simulink model "SpringMass_Model_SDomain"  (R2020a)
settings: Solver=VariableStepAuto  StartTime=0.0  StopTime=10  MaxStep=0.05  RelTol=1e-3
values from neighbouring files (symbols this model uses):
  b = 1.8    [SpringMass_mScript_SDomain.m]    (also in SpringMass_mScript_TDomain.m = 2)
  F = 10    [SpringMass_mScript_SDomain.m]    (also in SpringMass_mScript_TDomain.m)
  k = 10    [SpringMass_mScript_SDomain.m]    (also in SpringMass_mScript_TDomain.m = 20)
  M = 1    [SpringMass_mScript_SDomain.m]    (also in SpringMass_mScript_TDomain.m)
settings Model: Creator=alexd  LastModifiedBy=alexd

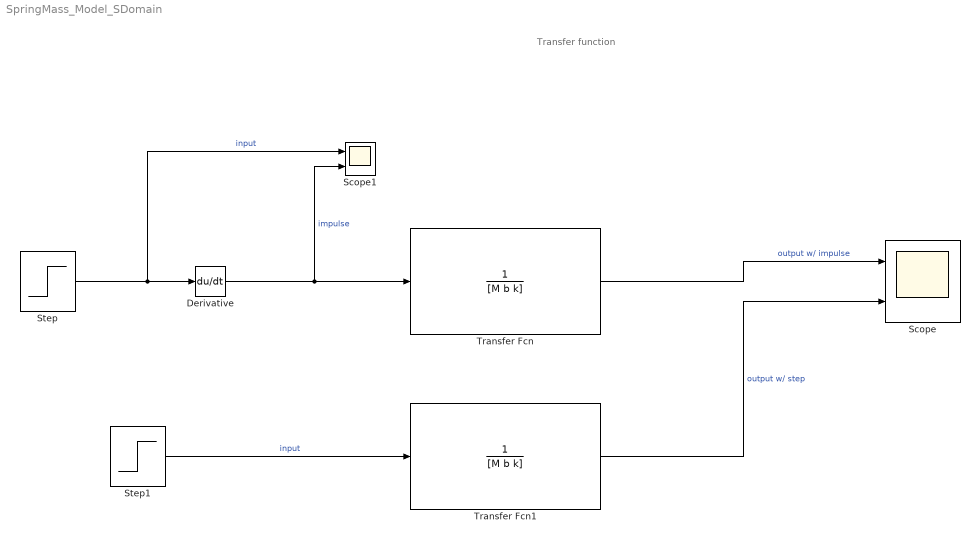
== system SpringMass_Model_SDomain ==
  note: Transfer function
  Derivative : Derivative
  Scope : Scope  NumInputPorts=2
  Scope1 : Scope  NumInputPorts=2
  Step : Step  After=F  SampleTime=0
  Step1 : Step  After=F  SampleTime=0
  Transfer Fcn : TransferFcn  Denominator=[M b k]
  Transfer Fcn1 : TransferFcn  Denominator=[M b k]
  wires:
  Transfer Fcn/1 -> Scope/1  "output w/ impulse"
  Step/1 -> Scope1/1, Derivative/1  "input"
  Derivative/1 -> Scope1/2, Transfer Fcn/1  "impulse"
  Transfer Fcn1/1 -> Scope/2  "output w/ step"
  Step1/1 -> Transfer Fcn1/1  "input"
